simulink model "f3forN4"  (R2016b)
settings: Solver=FixedStepDiscrete  StartTime=0.0  StopTime=10.0  RelTol=1e-3
libraries: simulink x6
settings Model: DataTypeOverride=Off  Creator=hasee  LastModifiedBy=hasee
settings DataIOCC: LimitDataPoints=on  SaveOutput=off  SaveTime=off
settings OptimizationCC: BlockReduction=off  ConditionallyExecuteInputs=off  DefaultParameterBehavior=Inlined  LifeSpan=inf
settings DebuggingCC: AlgebraicLoopMsg=error  SingleTaskRateTransMsg=error  AllowSymbolicDim=off  StrictBusMsg=ErrorOnBusTreatedAsVector  SFUnexpectedBacktrackingDiag=warning  SFNoUnconditionalDefaultTransitionDiag=warning  SFExecutionAtInitializationDiag=none
settings HardwareCC: ProdBitPerPointer=32  ProdBitPerSizeT=32  ProdBitPerPtrDiffT=32  ProdLargestAtomicFloat=None  ProdIntDivRoundTo=Undefined  ProdEndianess=Unspecified  ProdWordSize=32  ProdHWDeviceType=ASIC/FPGA->ASIC/FPGA  ProdEqTarget=off
settings GRTTargetCC: TargetLangStandard=C89/C90 (ANSI)  GeneratePreprocessorConditionals=Disable all
settings ConfigComp: CovScope=ReferencedModels  CovMetricSettings=dw  CovHtmlReporting=on  CovSaveCumulativeToWorkspaceVar=on  CovSaveSingleToWorkspaceVar=on  CovExternalEMLEnable=off  CovSFcnEnable=off

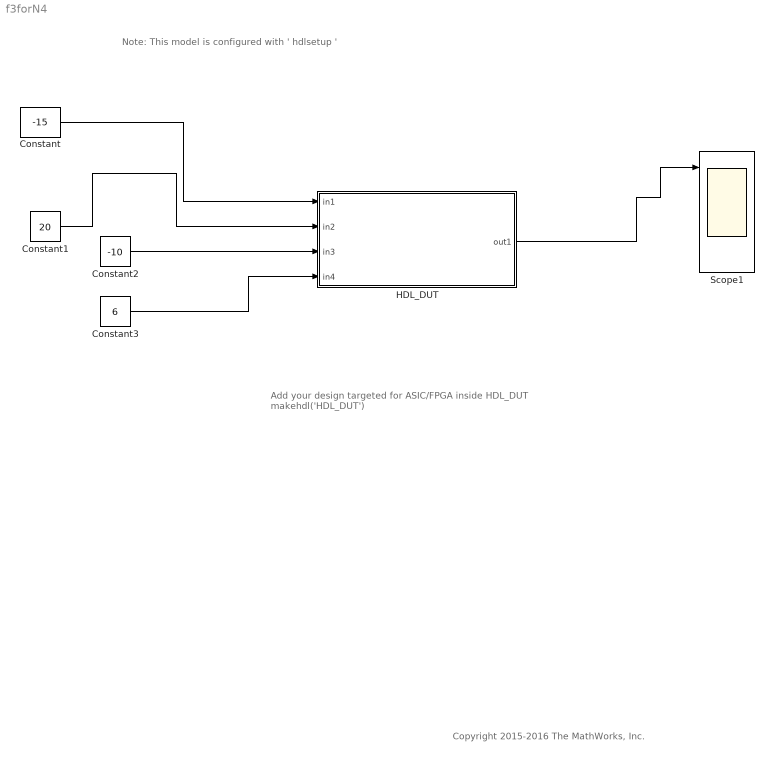
== system f3forN4 ==
  note: Note: This model is configured with ' hdlsetup '
  note: Add your design targeted for ASIC/FPGA inside HDL_DUT
      | makehdl('HDL_DUT')
  note: Copyright 2015-2016 The MathWorks, Inc.
  Constant : Constant  Value=-15  OutDataTypeStr=int8  SampleTime=-1
  Constant1 : Constant  Value=20  OutDataTypeStr=int8  SampleTime=-1
  Constant2 : Constant  Value=-10  OutDataTypeStr=int8  SampleTime=-1
  Constant3 : Constant  Value=6  OutDataTypeStr=int8  SampleTime=-1
  HDL_DUT : Subsystem
  Scope1 : Scope  NumInputPorts=4
  wires:
  HDL_DUT/1(out1) -> Scope1/1
  Constant1/1 -> HDL_DUT/2(in2)
  Constant/1 -> HDL_DUT/1(in1)
  Constant2/1 -> HDL_DUT/3(in3)
  Constant3/1 -> HDL_DUT/4(in4)

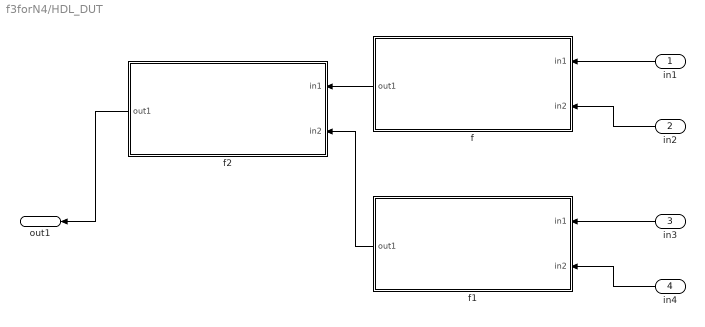
== system f3forN4/HDL_DUT ==
  in1 : Inport  OutDataTypeStr=int8
  in2 : Inport  Port=2  OutDataTypeStr=int8
  in3 : Inport  Port=3  OutDataTypeStr=int8
  in4 : Inport  Port=4  OutDataTypeStr=int8
  f : Subsystem
  f1 : Subsystem
  f2 : Subsystem
  out1 : Outport
  wires:
  in1/1 -> f/1(in1)
  in2/1 -> f/2(in2)
  in3/1 -> f1/1(in1)
  in4/1 -> f1/2(in2)
  f/1(out1) -> f2/1(in1)
  f1/1(out1) -> f2/2(in2)
  f2/1(out1) -> out1/1

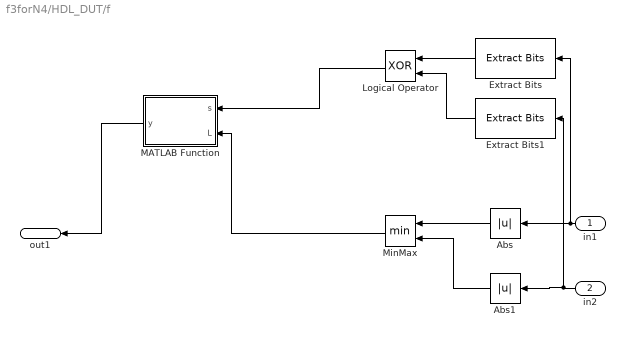
== system f3forN4/HDL_DUT/f ==
  in1 : Inport  OutDataTypeStr=int8
  in2 : Inport  Port=2  OutDataTypeStr=int8
  Abs : Abs
  Abs1 : Abs
  Extract Bits : simulink/Logic and Bit Operations/Extract Bits  bitsToExtract=Range starting with most significant bit  numBits=1  bitIdxRange=[0 ]  outScalingMode=Preserve fixed-point scaling
  Extract Bits1 : simulink/Logic and Bit Operations/Extract Bits  bitsToExtract=Range starting with most significant bit  numBits=1  bitIdxRange=[0 ]  outScalingMode=Preserve fixed-point scaling
  Logical Operator : Logic  Operator=XOR  AllPortsSameDT=off  OutDataTypeStr=boolean
  MATLAB Function : MATLAB Function  TreatAsAtomicUnit=on
  MinMax : MinMax  Inputs=2
  out1 : Outport
  wires:
  Extract Bits/1 -> Logical Operator/1
  in1/1 -> Abs/1, Extract Bits/1
  in2/1 -> Abs1/1, Extract Bits1/1
  Extract Bits1/1 -> Logical Operator/2
  Logical Operator/1 -> MATLAB Function/1(s)
  Abs/1 -> MinMax/1
  Abs1/1 -> MinMax/2
  MinMax/1 -> MATLAB Function/2(L)
  MATLAB Function/1(y) -> out1/1

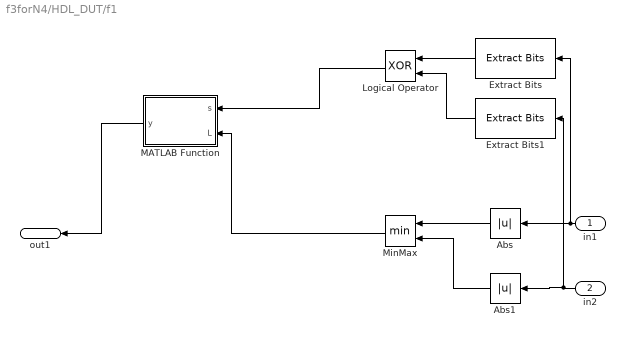
== system f3forN4/HDL_DUT/f1 ==
  in1 : Inport  OutDataTypeStr=int8
  in2 : Inport  Port=2  OutDataTypeStr=int8
  Abs : Abs
  Abs1 : Abs
  Extract Bits : simulink/Logic and Bit Operations/Extract Bits  bitsToExtract=Range starting with most significant bit  numBits=1  bitIdxRange=[0 ]  outScalingMode=Preserve fixed-point scaling
  Extract Bits1 : simulink/Logic and Bit Operations/Extract Bits  bitsToExtract=Range starting with most significant bit  numBits=1  bitIdxRange=[0 ]  outScalingMode=Preserve fixed-point scaling
  Logical Operator : Logic  Operator=XOR  AllPortsSameDT=off  OutDataTypeStr=boolean
  MATLAB Function : MATLAB Function  TreatAsAtomicUnit=on
  MinMax : MinMax  Inputs=2
  out1 : Outport
  wires:
  Extract Bits/1 -> Logical Operator/1
  in1/1 -> Abs/1, Extract Bits/1
  in2/1 -> Abs1/1, Extract Bits1/1
  Extract Bits1/1 -> Logical Operator/2
  Logical Operator/1 -> MATLAB Function/1(s)
  Abs/1 -> MinMax/1
  Abs1/1 -> MinMax/2
  MinMax/1 -> MATLAB Function/2(L)
  MATLAB Function/1(y) -> out1/1

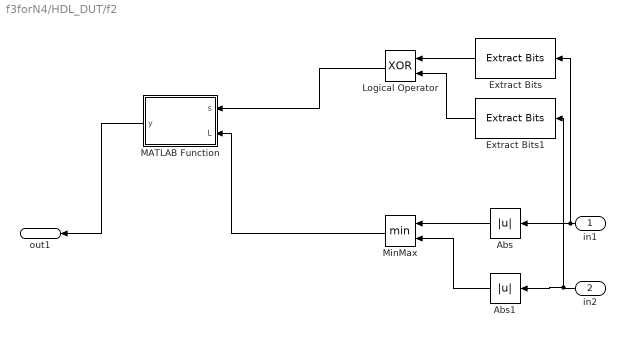
== system f3forN4/HDL_DUT/f2 ==
  in1 : Inport  OutDataTypeStr=int8
  in2 : Inport  Port=2  OutDataTypeStr=int8
  Abs : Abs
  Abs1 : Abs
  Extract Bits : simulink/Logic and Bit Operations/Extract Bits  bitsToExtract=Range starting with most significant bit  numBits=1  bitIdxRange=[0 ]  outScalingMode=Preserve fixed-point scaling
  Extract Bits1 : simulink/Logic and Bit Operations/Extract Bits  bitsToExtract=Range starting with most significant bit  numBits=1  bitIdxRange=[0 ]  outScalingMode=Preserve fixed-point scaling
  Logical Operator : Logic  Operator=XOR  AllPortsSameDT=off  OutDataTypeStr=boolean
  MATLAB Function : MATLAB Function  TreatAsAtomicUnit=on
  MinMax : MinMax  Inputs=2
  out1 : Outport
  wires:
  Extract Bits/1 -> Logical Operator/1
  in1/1 -> Abs/1, Extract Bits/1
  in2/1 -> Abs1/1, Extract Bits1/1
  Extract Bits1/1 -> Logical Operator/2
  Logical Operator/1 -> MATLAB Function/1(s)
  Abs/1 -> MinMax/1
  Abs1/1 -> MinMax/2
  MinMax/1 -> MATLAB Function/2(L)
  MATLAB Function/1(y) -> out1/1

== matlab function f3forN4/HDL_DUT/f/MATLAB Function ==
  data: s input; y output; L input
function y = fcn(s,L)
%#codegen
if s ==1
    y = -L;
else
    y = L;
end

== matlab function f3forN4/HDL_DUT/f1/MATLAB Function ==
  data: s input; y output; L input
function y = fcn(s,L)
%#codegen
if s ==1
    y = -L;
else
    y = L;
end

== matlab function f3forN4/HDL_DUT/f2/MATLAB Function ==
  data: s input; y output; L input
function y = fcn(s,L)
%#codegen
if s ==1
    y = -L;
else
    y = L;
end
